simulink model "Furuta_Template"  (Simulink 9.0)
settings: Solver=ode1  StartTime=0.0  StopTime=30  FixedStep=0.001  RelTol=1e-8  EnableMultiTasking=on
values from neighbouring files (symbols this model uses):
  A1 = -b1*J2    (= -5.5328e-07)    [Furuta233.m]    (also in Furuta_.m; Furuta_Template.m; Real_parameters.m = -2.0831968e-07)
  A2 = m2*L1*l2*b2    (= 8.64024e-07)    [Furuta233.m]    (also in Furuta_.m; Furuta_Template.m; Real_parameters.m = m2*L1*l2*b2)
  A3 = -((J2)^2)    (= -3.061187584e-05)    [Furuta233.m]    (also in Furuta_.m; Furuta_Template.m; Real_parameters.m = -4.33970890753e-06)
  A4 = -0.5*((J2)^2)*m2*L1*l2    (= -4.72310632335e-08)    [Furuta233.m]    (also in Furuta_.m; Furuta_Template.m = -0.5*((J2)^2*m2*L1*l2; Real_parameters.m = -0.5*((J2)^2)*m2*L1*l2)
  A5 = J2*m2*L1*l2    (= 1.707311424e-05)    [Furuta233.m]    (also in Furuta_.m; Furuta_Template.m; Real_parameters.m = J2*m2*L1*l2)
  A6 = J2    (= 0.0055328)    [Furuta233.m]    (also in Furuta_.m; Furuta_Template.m; Real_parameters.m = 0.0020831968)
  A7 = -m2*L1*l2    (= -0.0030858)    [Furuta233.m]    (also in Furuta_.m; Furuta_Template.m; Real_parameters.m = -m2*L1*l2)
  A8 = 0.5*((m2)^2)*((l2)^2)*(L1)    (= 1.712619e-05)    [Furuta233.m]    (also in Furuta_.m = 3.796875e-05; Furuta_Template.m = 3.796875e-05; Real_parameters.m = 0.5*((m2)^2)*((l2)^2)*(L1))
  A_MAT = [0 0 1 0;0 0 0 1;A31 A32 A33 A34;A41 A42 A43 A44]    [Furuta233.m]    (also in Furuta_.m = [0 0 1 0;0 0 0 1;0 H1 H2 H3;0 H4 H5 H6]; Furuta_Template.m = [0 0 1 0;0 0 0 1;0 H1 H2 H3;0 H4 H5 H6]; Real_parameters.m = [0 0 1 0;0 0 0 1;0 24.4662 -0.0062 -0.0664;0 65.7367 -0.0051)
  B1 = m2*L1*l2*b1    (= 3.0858e-07)    [Furuta233.m]    (also in Furuta_.m; Furuta_Template.m; Real_parameters.m = m2*L1*l2*b1)
  B10 = J2    (= 0.0055328)    [Furuta233.m]    (also in Furuta_.m; Furuta_Template.m; Real_parameters.m = 0.0020831968)
  B11 = -m2*l2*J0    (= -0.00041454393)    [Furuta233.m]    (also in Furuta_.m; Furuta_Template.m; Real_parameters.m = -m2*l2*J0)
  B12 = -m2*l2*J2    (= -6.141408e-05)    [Furuta233.m]    (also in Furuta_.m; Furuta_Template.m; Real_parameters.m = -m2*l2*J2)
  B2 = -J0*b2    (= -1.0456964e-05)    [Furuta233.m]    (also in Furuta_.m; Furuta_Template.m; Real_parameters.m = -1.40929954668e-06)
  B3 = -J2*b2    (= -1.549184e-06)    [Furuta233.m]    (also in Furuta_.m; Furuta_Template.m; Real_parameters.m = -5.83295104e-07)
  B4 = m2*L1*l2*J2    (= 1.707311424e-05)    [Furuta233.m]    (also in Furuta_.m; Furuta_Template.m; Real_parameters.m = m2*L1*l2*J2)
  B5 = 0.5*J0*J2    (= 0.00010331480432)    [Furuta233.m]    (also in Furuta_.m; Furuta_Template.m; Real_parameters.m = 5.24258626052e-06)
  B6 = 0.5*((J2)^2)    (= 1.530593792e-05)    [Furuta233.m]    (also in Furuta_.m; Furuta_Template.m = 0.5*((j2)^2); Real_parameters.m = 2.16985445377e-06)
  B7 = -0.5*((m2)^2)*((L1)^2)*((l2)^2)    (= -4.76108082e-06)    [Furuta233.m]    (also in Furuta_.m; Furuta_Template.m; Real_parameters.m = -0.5*((m2)^2)*((L1)^2)*((l2)^2))
  B8 = -m2*L1*l2    (= -0.0030858)    [Furuta233.m]    (also in Furuta_.m; Furuta_Template.m; Real_parameters.m = -m2*L1*l2)
  B9 = J0    (= 0.0373463)    [Furuta233.m]    (also in Furuta_.m; Furuta_Template.m; Real_parameters.m = 0.00503321266673)
  B_MAT = [0;0;B31;B41]    [Furuta233.m]    (also in Furuta_.m = [0;0;H7;H8]; Furuta_Template.m = [0;0;H7;H8]; Real_parameters.m = [0;0;3.2;3.1])
  C1 = -km/Lm    (= -18)    [Furuta233.m]    (also in Furuta_.m = -km/Lm; Furuta_Template.m = -km/Lm; Real_parameters.m)
  C2 = -Rm/Lm    (= -1560)    [Furuta233.m]    (also in Furuta_.m = -Rm/Lm; Furuta_Template.m = -Rm/Lm; Real_parameters.m)
  C3 = 1/Lm    (= 200)    [Furuta233.m]    (also in Furuta_.m = 1/Lm; Furuta_Template.m = 1/Lm; Real_parameters.m)
  C4 = km    (= 0.09)    [Furuta233.m]    (also in Furuta_.m = Km; Furuta_Template.m = Km; Real_parameters.m)
  C_MAT = [1 0 0 0;0 1 0 0]    [Furuta233.m]    (also in Furuta_.m = [1 1 0 0]; Furuta_Template.m = [1 1 0 0]; Real_parameters.m)
  D1 = J0*J2    (= 0.00020662960864)    [Furuta233.m]    (also in Furuta_.m; Furuta_Template.m; Real_parameters.m = 1.0485172521e-05)
  D2 = (J2)^2    (= 3.061187584e-05)    [Furuta233.m]    (also in Furuta_.m; Furuta_Template.m; Real_parameters.m = 4.33970890753e-06)
  D3 = ((m2)^2)*((L1)^2)*((l2)^2)    (= 9.52216164e-06)    [Furuta233.m]    (also in Furuta_.m; Furuta_Template.m; Real_parameters.m = ((m2)^2)*((L1)^2)*((l2)^2))
  E0 = 0.05    [Furuta233.m]    (also in Real_parameters.m = 0)
  F_MAT = -lqr(A_MAT,B_MAT,Q,R)    [Furuta233.m]    (also in Real_parameters.m = -[0.16 -320 1.3 -16])
  g = 9.81    [Furuta233.m]    (also in Furuta_.m; Furuta_Template.m; Real_parameters.m)
  J2 = J2_1+(m2*((l2)^2))    (= 0.0055328)    [Furuta233.m]    (also in Furuta_.m; Furuta_Template.m; Real_parameters.m = 0.0020831968)
  K_swing = 0.1    [Furuta233.m]    (also in Real_parameters.m = -100)
  l2 = 0.148    [Furuta233.m]    (also in Furuta_.m; Furuta_Template.m; Real_parameters.m = sqrt(J2/m2))
  L_MAT = -place(A_MAT',C_MAT',10*Closed_Loop_Poles)'    [Furuta233.m]    (also in Real_parameters.m = place(A_MAT',C_MAT',[12*Closed_Loop_Poles(1) 12*Closed_Loop_)
  m2 = 0.075    [Furuta233.m]    (also in Furuta_.m; Furuta_Template.m; Real_parameters.m = 0.049)
settings Model: Creator=mecmg  LastModifiedBy=lenovo
settings DataIOCC: LimitDataPoints=on
settings OptimizationCC: ExpressionDepthLimit=2147483647
settings DebuggingCC: SolverPrmCheckMsg=warning  FcnCallInpInsideContextMsg=warning  StateNameClashWarn=warning
settings GRTTargetCC: GeneratePreprocessorConditionals=Disable all  CombineOutputUpdateFcns=off  GRTInterface=on

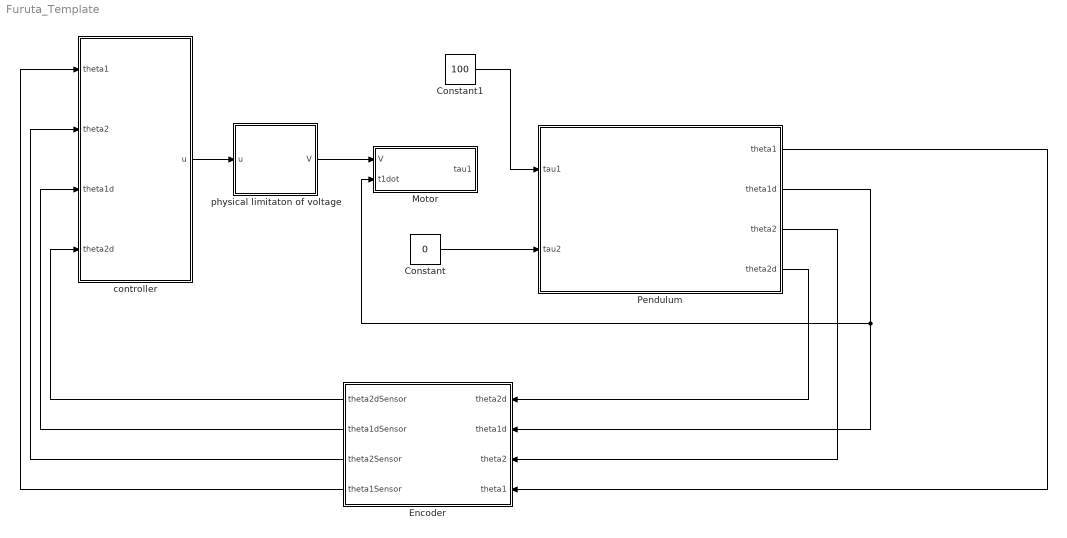
== system Furuta_Template ==
  Constant : Constant  Value=0  VectorParams1D=off
  Constant1 : Constant  Value=100
  Encoder : Subsystem
  Motor : Subsystem
  Pendulum : Subsystem
  controller : Subsystem
  physical limitaton of voltage : Subsystem
  wires:
  controller/1(u) -> physical limitaton of voltage/1(u)
  Encoder/1(theta2dSensor) -> controller/4(theta2d)
  Encoder/4(theta1Sensor) -> controller/1(theta1)
  Encoder/2(theta1dSensor) -> controller/3(theta1d)
  Encoder/3(theta2Sensor) -> controller/2(theta2)
  Pendulum/4(theta2d) -> Encoder/1(theta2d)
  Constant/1 -> Pendulum/2(tau2)
  Pendulum/1(theta1) -> Encoder/4(theta1)
  Pendulum/3(theta2) -> Encoder/3(theta2)
  Pendulum/2("theta1d ") -> Motor/2(t1dot), Encoder/2(theta1d)
  physical limitaton of voltage/1(V) -> Motor/1(V)
  Constant1/1 -> Pendulum/1(tau1)

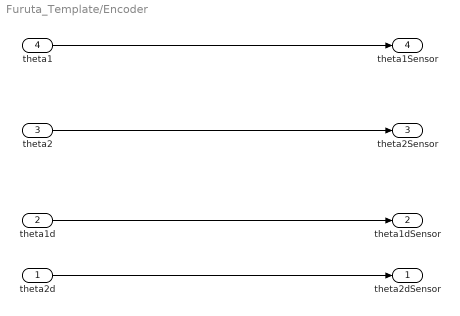
== system Furuta_Template/Encoder ==
  theta2d : Inport
  theta1d : Inport  Port=2
  theta2 : Inport  Port=3
  theta1 : Inport  Port=4
  theta2dSensor : Outport
  theta1dSensor : Outport  Port=2
  theta2Sensor : Outport  Port=3
  theta1Sensor : Outport  Port=4
  wires:
  theta1/1 -> theta1Sensor/1
  theta2/1 -> theta2Sensor/1
  theta1d/1 -> theta1dSensor/1
  theta2d/1 -> theta2dSensor/1

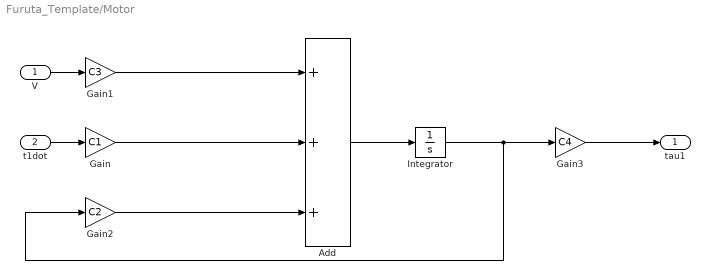
== system Furuta_Template/Motor ==
  V : Inport
  t1dot : Inport  Port=2
  Add : Sum  Inputs=+++
  Gain : Gain  Gain=C1
  Gain1 : Gain  Gain=C3
  Gain2 : Gain  Gain=C2
  Gain3 : Gain  Gain=C4
  Integrator : Integrator
  tau1 : Outport
  wires:
  t1dot/1 -> Gain/1
  Gain1/1 -> Add/1
  Gain/1 -> Add/2
  Gain2/1 -> Add/3
  Add/1 -> Integrator/1
  Integrator/1 -> Gain3/1, Gain2/1
  Gain3/1 -> tau1/1
  V/1 -> Gain1/1

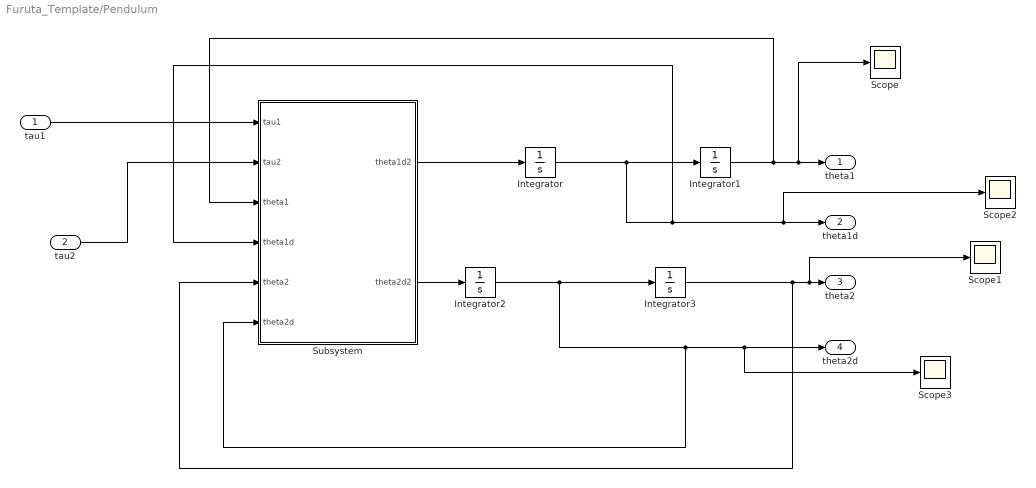
== system Furuta_Template/Pendulum ==
  tau1 : Inport
  tau2 : Inport  Port=2
  Integrator : Integrator
  Integrator1 : Integrator
  Integrator2 : Integrator
  Integrator3 : Integrator  InitialCondition=190/180*pi
  Scope{,1..3} (4 alike) : Scope
  Subsystem : Subsystem
  theta1 : Outport
  "theta1d " : Outport  Port=2
  theta2 : Outport  Port=3
  theta2d : Outport  Port=4
  wires:
  Subsystem/1(theta1d2) -> Integrator/1
  Integrator2/1 -> Subsystem/6(theta2d), Scope3/1, theta2d/1, Integrator3/1
  Integrator3/1 -> Scope1/1, theta2/1, Subsystem/5(theta2)
  Integrator/1 -> Integrator1/1, Scope2/1, "theta1d "/1, Subsystem/4(theta1d)
  Integrator1/1 -> Subsystem/3(theta1), Scope/1, theta1/1
  Subsystem/2(theta2d2) -> Integrator2/1
  tau1/1 -> Subsystem/1(tau1)
  tau2/1 -> Subsystem/2(tau2)

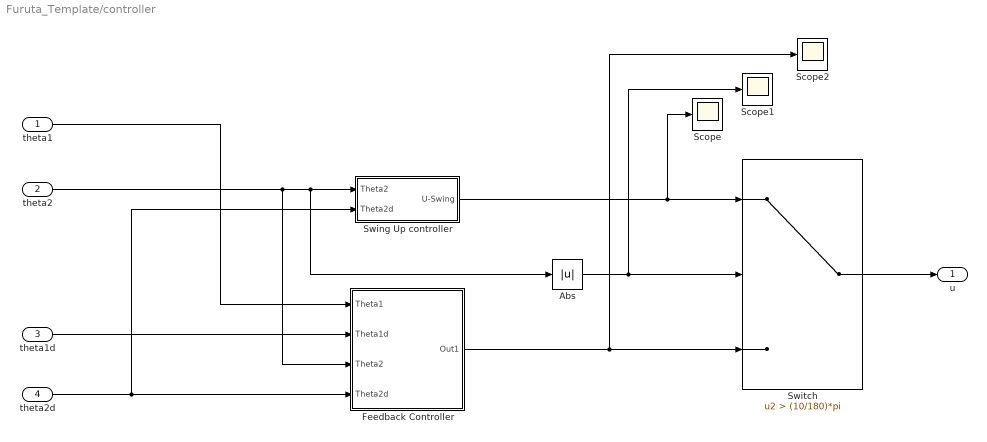
== system Furuta_Template/controller ==
  theta1 : Inport
  theta2 : Inport  Port=2
  theta1d : Inport  Port=3
  theta2d : Inport  Port=4
  Abs : Abs
  Feedback Controller : Subsystem
  Scope : Scope
  Scope1 : Scope
  Scope2 : Scope
  Swing Up controller : Subsystem
  Switch : Switch  Criteria=u2 > Threshold  Threshold=(10/180)*pi
  u : Outport
  wires:
  theta2/1 -> Feedback Controller/3(Theta2), Abs/1, Swing Up controller/1("Theta2 ")
  theta1/1 -> Feedback Controller/1("Theta1 ")
  theta1d/1 -> Feedback Controller/2("Theta1d ")
  theta2d/1 -> Swing Up controller/2("Theta2d "), Feedback Controller/4("Theta2d ")
  Feedback Controller/1(Out1) -> Scope2/1, Switch/3
  Abs/1 -> Scope1/1, Switch/2
  Switch/1 -> u/1
  Swing Up controller/1("U-Swing ") -> Scope/1, Switch/1

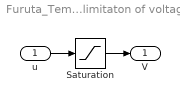
== system Furuta_Template/physical limitaton of voltage ==
  u : Inport
  Saturation : Saturate  UpperLimit=10  LowerLimit=-10
  V : Outport
  wires:
  u/1 -> Saturation/1
  Saturation/1 -> V/1

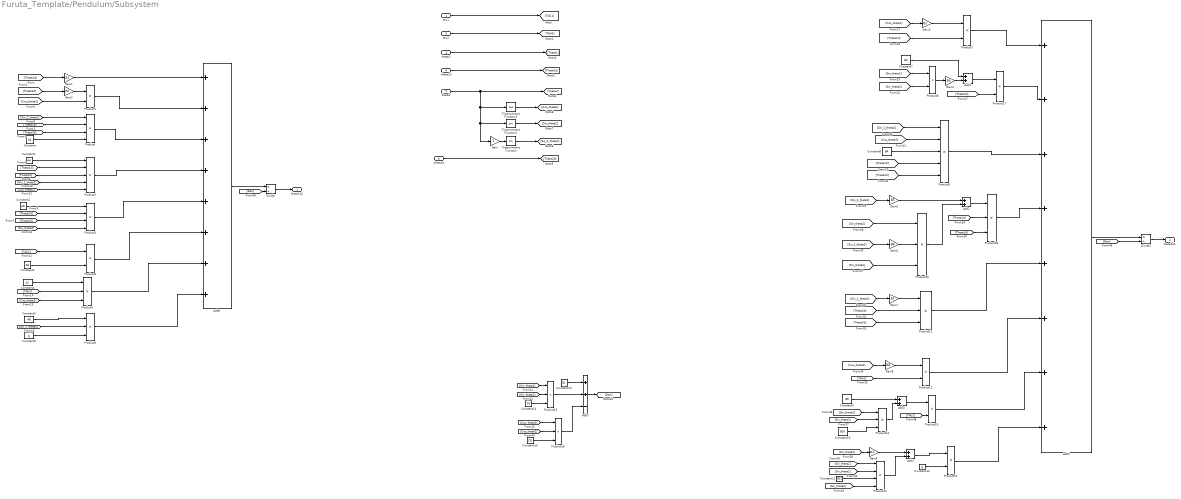
== system Furuta_Template/Pendulum/Subsystem ==
  tau1 : Inport
  tau2 : Inport  Port=2
  theta1 : Inport  Port=3
  theta1d : Inport  Port=4
  theta2 : Inport  Port=5
  theta2d : Inport  Port=6
  Add{1..4} (4 alike) : Sum
  Add5 : Sum  Inputs=++++++++
  Add6 : Sum  Inputs=++++++++
  Add7 : Sum  Inputs=++-
  Constant : Constant  Value=A3
  Constant1 : Constant  Value=A4
  Constant10 : Constant  Value=B10
  Constant11 : Constant  Value=B12
  Constant12 : Constant  Value=g
  Constant13 : Constant  Value=D1
  Constant14 : Constant  Value=D2
  Constant15 : Constant  Value=D3
  Constant2 : Constant  Value=A5
  Constant3 : Constant  Value=A6
  Constant4 : Constant  Value=A7
  Constant5 : Constant  Value=A8
  Constant6 : Constant  Value=g
  Constant7 : Constant  Value=B2
  Constant8 : Constant  Value=B4
  Constant9 : Constant  Value=B9
  Divide : Product  Inputs=*/
  Divide1 : Product  Inputs=*/
  Gain : Gain  Gain=2
  Gain1 : Gain  Gain=A1
  Gain2 : Gain  Gain=A2
  Gain3 : Gain  Gain=B1
  Gain4 : Gain  Gain=B3
  Gain5 : Gain  Gain=B5
  Gain6 : Gain  Gain=B6
  Gain7 : Gain  Gain=B7
  Gain8 : Gain  Gain=B8
  Gain9 : Gain  Gain=B11
  Product : Product  Inputs=4
  Product{1,4,7..8,12,17,19..20} (8 alike) : Product
  Product{5..6,10..11,13,15..16,18} (8 alike) : Product  Inputs=3
  Product14 : Product  Inputs=4
  Product2 : Product  Inputs=5
  Product3 : Product  Inputs=4
  Product9 : Product  Inputs=5
  Trigonometric Function : Trigonometry
  Trigonometric Function1 : Trigonometry
  Trigonometric Function2 : Trigonometry  Operator=cos
  theta1d2 : Outport
  theta2d2 : Outport  Port=2
  wires:
  tau2/1 -> [TAU2]
  tau1/1 -> [TAU1]
  theta1/1 -> [Theta1]
  theta1d/1 -> [Theta1d]
  theta2/1 -> [Theta2], Trigonometric Function2/1, Trigonometric Function1/1, Gain/1
  theta2d/1 -> [Theta2d]
  Trigonometric Function1/1 -> [Sin_theta2]
  Gain/1 -> Trigonometric Function/1
  Trigonometric Function2/1 -> [Cos_theta2]
  Trigonometric Function/1 -> [Sin_2_theta2]
  [Cos_theta2] -> Gain3/1
  [Sin_2_theta2] -> Gain6/1
  Gain3/1 -> Product7/1
  Gain8/1 -> Product12/1
  Product9/1 -> Add5/3
  Constant9/1 -> Add3/1
  [Theta2d] -> Product9/5
  [Sin_theta2] -> Gain9/1
  Gain9/1 -> Add4/1
  [Theta1d] -> Product7/2
  Constant8/1 -> Product9/3
  Product12/1 -> Add5/6
  [Sin_theta2] -> Product13/2
  Gain7/1 -> Product11/1
  [Cos_theta2] -> Gain8/1
  Product7/1 -> Add5/1
  Product14/1 -> Add4/2
  [Sin_2_theta2] -> Gain7/1
  [Sin_theta2] -> Product14/2
  Product8/1 -> Gain4/1
  [Theta1d] -> Product9/4
  Product11/1 -> Add5/5
  [Sin_theta2] -> Product8/1
  [Sin_theta2] -> Product10/3
  Constant7/1 -> Add1/1
  [Theta2d] -> Product11/3
  [Cos_theta2] -> Product9/2
  Gain6/1 -> Product10/2
  Gain5/1 -> Add2/1
  [Sin_2_theta2] -> Gain5/1
  Gain4/1 -> Add1/2
  [Sin_theta2] -> Product10/1
  [TAU1] -> Product12/2
  [Sin_theta2] -> Product14/4
  Constant11/1 -> Product14/3
  Product10/1 -> Add2/2
  [Sin_theta2] -> Product13/1
  [Theta2d] -> Product11/2
  [Sin_theta2] -> Product14/1
  Constant10/1 -> Product13/3
  [Sin_theta2] -> Product8/2
  Divide/1 -> theta1d2/1
  Product6/1 -> Add6/8
  Constant5/1 -> Product6/1
  [Den] -> Divide/2
  Add6/1 -> Divide/1
  [Cos_theta2] -> Product1/2
  [Cos_theta2] -> Product2/5
  [TAU2] -> Product5/2
  [Sin_2_theta2] -> Product6/2
  Product3/1 -> Add6/5
  Product1/1 -> Add6/2
  Constant4/1 -> Product5/1
  Product/1 -> Add6/3
  Constant1/1 -> Product2/1
  Constant2/1 -> Product3/1
  Constant3/1 -> Product4/2
  Gain2/1 -> Product1/1
  Constant/1 -> Product/4
  [Sin_2_theta2] -> Product2/4
  [Theta2d] -> Product3/2
  Constant6/1 -> Product6/3
  [Theta1d] -> Gain1/1
  [Theta2d] -> Product/3
  [Sin_2_theta2] -> Product/1
  [Cos_theta2] -> Product5/3
  Gain1/1 -> Add6/1
  [Sin_theta2] -> Product3/4
  [Theta1d] -> Product2/3
  [Theta1d] -> Product2/2
  [Theta2d] -> Gain2/1
  Product2/1 -> Add6/4
  [Theta1d] -> Product/2
  [Theta2d] -> Product3/3
  Product4/1 -> Add6/6
  [TAU1] -> Product4/1
  Product5/1 -> Add6/7
  Constant15/1 -> Product16/3
  [Sin_theta2] -> Product15/2
  [Cos_theta2] -> Product16/1
  Product16/1 -> Add7/3
  [Sin_theta2] -> Product15/1
  Constant14/1 -> Product15/3
  [Cos_theta2] -> Product16/2
  Constant13/1 -> Add7/1
  Add7/1 -> [Den]
  Product15/1 -> Add7/2
  Add1/1 -> Product17/1
  Product17/1 -> Add5/2
  [Theta2d] -> Product17/2
  [Sin_2_theta2] -> Product9/1
  Add2/1 -> Product18/1
  [Theta1d] -> Product18/2
  Product18/1 -> Add5/4
  Add3/1 -> Product19/1
  [TAU2] -> Product19/2
  Product19/1 -> Add5/7
  Product13/1 -> Add3/2
  Add4/1 -> Product20/1
  Constant12/1 -> Product20/2
  Product20/1 -> Add5/8
  [Theta1d] -> Product18/3
  [Den] -> Divide1/2
  Add5/1 -> Divide1/1
  Divide1/1 -> theta2d2/1

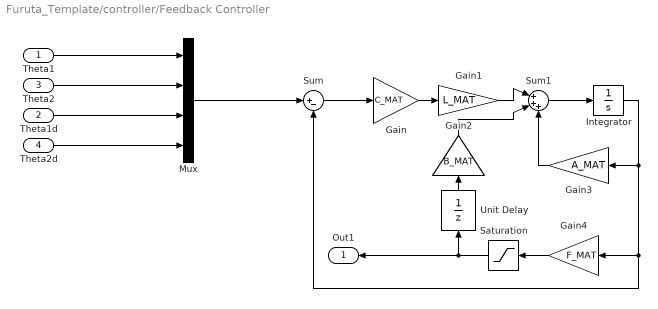
== system Furuta_Template/controller/Feedback Controller ==
  "Theta1 " : Inport
  "Theta1d " : Inport  Port=2
  Theta2 : Inport  Port=3
  "Theta2d " : Inport  Port=4
  Gain : Gain  Gain=C_MAT
  Gain1 : Gain  Gain=L_MAT
  Gain2 : Gain  Gain=B_MAT
  Gain3 : Gain  Gain=A_MAT
  Gain4 : Gain  Gain=F_MAT
  Integrator : Integrator
  Mux : Mux
  Saturation : Saturate
  Sum : Sum  Inputs=|+-
  Sum1 : Sum  Inputs=|+++
  Unit Delay : UnitDelay  SampleTime=-1
  Out1 : Outport
  wires:
  "Theta1 "/1 -> Mux/1
  Theta2/1 -> Mux/2
  "Theta1d "/1 -> Mux/3
  "Theta2d "/1 -> Mux/4
  Mux/1 -> Sum/1
  Sum/1 -> Gain/1
  Gain/1 -> Gain1/1
  Sum1/1 -> Integrator/1
  Gain1/1 -> Sum1/1
  Gain2/1 -> Sum1/2
  Integrator/1 -> Sum/2, Gain4/1, Gain3/1
  Gain3/1 -> Sum1/3
  Gain4/1 -> Saturation/1
  Saturation/1 -> Unit Delay/1, Out1/1
  Unit Delay/1 -> Gain2/1

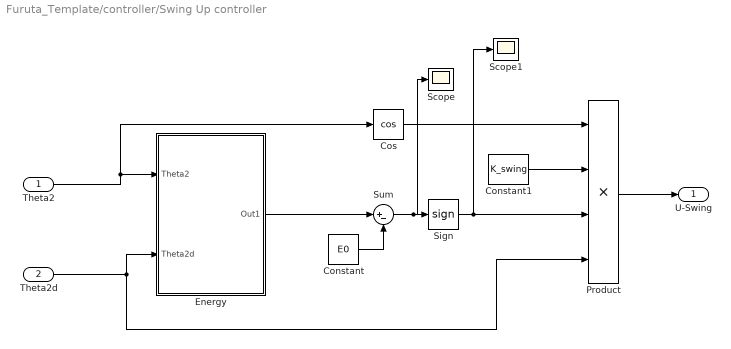
== system Furuta_Template/controller/Swing Up controller ==
  "Theta2 " : Inport
  "Theta2d " : Inport  Port=2
  Constant : Constant  Value=E0
  Constant1 : Constant  Value=K_swing
  Cos : Trigonometry  Operator=cos
  Energy : Subsystem
  Product : Product  Inputs=4
  Scope : Scope
  Scope1 : Scope
  Sign : Signum
  Sum : Sum  Inputs=|+-
  "U-Swing " : Outport
  wires:
  "Theta2 "/1 -> Cos/1, Energy/1("Theta2 ")
  "Theta2d "/1 -> Energy/2("Theta2d "), Product/4
  Energy/1(Out1) -> Sum/1
  Cos/1 -> Product/1
  Constant/1 -> Sum/2
  Sum/1 -> Scope/1, Sign/1
  Sign/1 -> Scope1/1, Product/3
  Constant1/1 -> Product/2
  Product/1 -> "U-Swing "/1

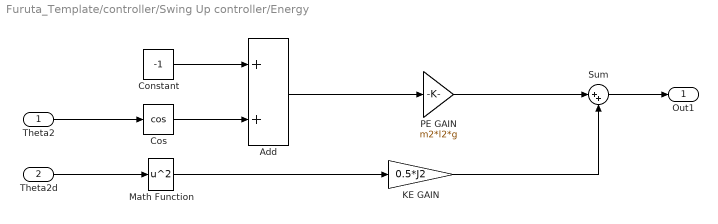
== system Furuta_Template/controller/Swing Up controller/Energy ==
  "Theta2 " : Inport
  "Theta2d " : Inport  Port=2
  Add : Sum
  Constant : Constant  Value=-1
  Cos : Trigonometry  Operator=cos
  KE GAIN : Gain  Gain=0.5*J2
  Math Function : Math  Operator=square  SaturateOnIntegerOverflow=on
  PE GAIN : Gain  Gain=m2*l2*g
  Sum : Sum  Inputs=|++
  Out1 : Outport
  wires:
  "Theta2 "/1 -> Cos/1
  Constant/1 -> Add/1
  Cos/1 -> Add/2
  Add/1 -> PE GAIN/1
  "Theta2d "/1 -> Math Function/1
  PE GAIN/1 -> Sum/1
  Math Function/1 -> KE GAIN/1
  KE GAIN/1 -> Sum/2
  Sum/1 -> Out1/1
